simulink library "ADV_BF_MASTERbak"  (Simulink 8.6)
settings: Solver=VariableStepAuto  StartTime=0.0  StopTime=10.0  RelTol=1e-3
libraries: cdsEpicsOut x30, cdsFilt x17, cdsFiltCtrl x14, cdsTP x14, cdsEpicsIn x7, cdsMuxMatrix x3, VIS_LIB x2, cdsOsc x1, cdsEpicsBinIn x1, cdsFunctionCall x1, SIXOSEM_F_STAGE_MASTER x1
(part 1 of 3)
settings Model: Creator=controls  LastModifiedBy=controls

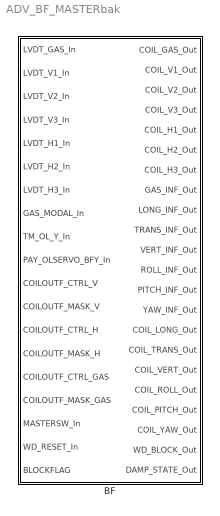
== system ADV_BF_MASTERbak ==
  BF : Subsystem

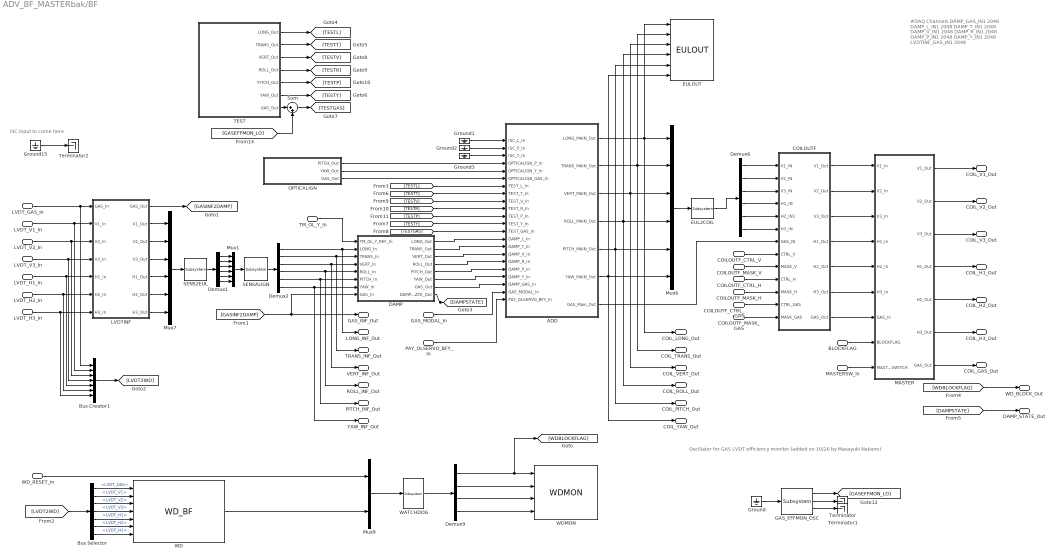
== system ADV_BF_MASTERbak/BF ==
  note: #DAQ Channels
      | DAMP_GAS_IN1 2048
      | DAMP_L_IN1 2048
      | DAMP_T_IN1 2048
      | DAMP_V_IN1 2048
      | DAMP_R_IN1 2048
      | DAMP_P_IN1 2048
      | DAMP_Y_IN1 2048
      | LVDTINF_GAS_IN1 2048
  note: ISC input to come here
  note: Oscillator for GAS LVDT efficiency monitor (added on 10/26 by Masayuki Nakano)
  LVDT_GAS_In : Inport
  LVDT_V1_In : Inport  Port=2
  LVDT_V2_In : Inport  Port=3
  LVDT_V3_In : Inport  Port=4
  LVDT_H1_In : Inport  Port=5
  LVDT_H2_In : Inport  Port=6
  LVDT_H3_In : Inport  Port=7
  GAS_MODAL_In : Inport  Port=8
  TM_OL_Y_In : Inport  Port=9
  PAY_OLSERVO_BFY_In : Inport  Port=10
  COILOUTF_CTRL_V : Inport  Port=11
  COILOUTF_MASK_V : Inport  Port=12
  COILOUTF_CTRL_H : Inport  Port=13
  COILOUTF_MASK_H : Inport  Port=14
  COILOUTF_CTRL_GAS : Inport  Port=15
  COILOUTF_MASK_GAS : Inport  Port=16
  MASTERSW_In : Inport  Port=17
  WD_RESET_In : Inport  Port=18
  BLOCKFLAG : Inport  Port=19
  ADD : Subsystem
  Bus Creator1 : BusCreator  Inputs='LVDT_GAS','LVDT_V1','LVDT_V2','LVDT_V3','LVDT_H1','LVDT_H2','LVDT_H3'
  Bus Selector : BusSelector  OutputSignals=LVDT_GAS,LVDT_V1,LVDT_V2,LVDT_V3,LVDT_H1,LVDT_H2,LVDT_H3
  COILOUTF : Subsystem
  DAMP : Subsystem
  Demux1 : Demux  Outputs=6
  Demux2 : Demux  Outputs=6
  Demux6 : Demux  Outputs=6
  Demux9 : Demux
  EUL2COIL : cdsMuxMatrix/Subsystem  Tag=cdsMuxMatrix  Description=|
      | ADL=SUS_INMATRIX.adl
      | SCRIPT=generate_KisselButton.py 4 5 #CHANNEL# > #TARGET_DIR#/#FULL_PART_NAME#_KB.adl
      settings: AttributesFormatString=%<Tag>
  EULOUT : VIS_LIB/EULOUT
  GAS_EFFMON_OSC : cdsOsc/Subsystem  Tag=cdsOsc  Description=Oscillator
      settings: AttributesFormatString=%<Tag>
  Ground{,1..3,15} (5 alike) : Ground
  LVDTINF : Subsystem
  MASTER : Subsystem
  Mux1 : Mux  Inputs=6
  Mux6 : Mux  Inputs=6
  Mux7 : Mux  Inputs=6
  Mux9 : Mux  Inputs=2
  OPTICALIGN : Subsystem
  SENS2EUL : cdsMuxMatrix/Subsystem  Tag=cdsMuxMatrix  Description=Any size matrix. Inputs and outputs must be connected using Mux and Demux parts.
      settings: AttributesFormatString=%<Tag>
  SENSALIGN : cdsMuxMatrix/Subsystem  Tag=cdsMuxMatrix  Description=Any size matrix. Inputs and outputs must be connected using Mux and Demux parts.
      settings: AttributesFormatString=%<Tag>
  Sum : Sum  Inputs=|++
  TEST : Subsystem
  Terminator : Terminator
  Terminator1 : Terminator
  Terminator2 : Terminator
  WATCHDOG : cdsFunctionCall/Subsystem  Tag=cdsFunctionCall  Description=inline OSEMWATCHDOG /opt/rtcds/userapps/release/vis/common/src/WATCHDOG.c
      settings: AttributesFormatString=%<Tag>\n%<Description>
  WD : VIS_LIB/WD_BF
  WDMON : SIXOSEM_F_STAGE_MASTER/SIXOSEM_F_STAGE_MASTER/WDMON
  COIL_GAS_Out : Outport
  COIL_V1_Out : Outport  Port=2
  COIL_V2_Out : Outport  Port=3
  COIL_V3_Out : Outport  Port=4
  COIL_H1_Out : Outport  Port=5
  COIL_H2_Out : Outport  Port=6
  COIL_H3_Out : Outport  Port=7
  GAS_INF_Out : Outport  Port=8
  LONG_INF_Out : Outport  Port=9
  TRANS_INF_Out : Outport  Port=10
  VERT_INF_Out : Outport  Port=11
  ROLL_INF_Out : Outport  Port=12
  PITCH_INF_Out : Outport  Port=13
  YAW_INF_Out : Outport  Port=14
  COIL_LONG_Out : Outport  Port=15
  COIL_TRANS_Out : Outport  Port=16
  COIL_VERT_Out : Outport  Port=17
  COIL_ROLL_Out : Outport  Port=18
  COIL_PITCH_Out : Outport  Port=19
  COIL_YAW_Out : Outport  Port=20
  WD_BLOCK_Out : Outport  Port=21
  DAMP_STATE_Out : Outport  Port=22
  wires:
  Ground15/1 -> Terminator2/1
  GAS_EFFMON_OSC/3 -> Terminator1/1
  GAS_EFFMON_OSC/2 -> Terminator/1
  Ground/1 -> GAS_EFFMON_OSC/1
  [GASEFFMON_LO] -> Sum/2
  Sum/1 -> [TESTGAS]
  TEST/7(GAS_Out) -> Sum/1
  GAS_EFFMON_OSC/1 -> [GASEFFMON_LO]
  COILOUTF_MASK_GAS/1 -> COILOUTF/13(MASK_GAS)
  COILOUTF_CTRL_GAS/1 -> COILOUTF/12(CTRL_GAS)
  COILOUTF_MASK_H/1 -> COILOUTF/11(MASK_H)
  COILOUTF_CTRL_H/1 -> COILOUTF/10(CTRL_H)
  LVDTINF/7(H3_Out) -> Mux7/6
  LVDTINF/6(H2_Out) -> Mux7/5
  LVDTINF/5(H1_Out) -> Mux7/4
  Bus Selector/7 -> WD/7  "<LVDT_H3>"
  Bus Selector/6 -> WD/6  "<LVDT_H2>"
  Bus Selector/5 -> WD/5  "<LVDT_H1>"
  Bus Selector/4 -> WD/4  "<LVDT_V3>"
  Bus Selector/3 -> WD/3  "<LVDT_V2>"
  Bus Selector/2 -> WD/2  "<LVDT_V1>"
  [DAMPSTATE] -> DAMP_STATE_Out/1
  [WDBLOCKFLAG] -> WD_BLOCK_Out/1
  MASTER/7(GAS_Out) -> COIL_GAS_Out/1
  MASTER/6(H3_Out) -> COIL_H3_Out/1
  MASTER/5(H2_Out) -> COIL_H2_Out/1
  MASTERSW_In/1 -> MASTER/9(MASTERSWITCH)
  BLOCKFLAG/1 -> MASTER/8(BLOCKFLAG)
  COILOUTF/4(H1_Out) -> MASTER/4(H1_In)
  COILOUTF/3(V3_Out) -> MASTER/3(V3_In)
  COILOUTF/2(V2_Out) -> MASTER/2(V2_In)
  COILOUTF/1(V1_Out) -> MASTER/1(V1_In)
  COILOUTF/7(GAS_Out) -> MASTER/7(GAS_In)
  COILOUTF/6(H3_Out) -> MASTER/6(H3_In)
  COILOUTF/5(H2_Out) -> MASTER/5(H2_In)
  Demux6/6 -> COILOUTF/6(H3_IN)
  Demux6/5 -> COILOUTF/5(H2_IN1)
  Demux6/4 -> COILOUTF/4(H1_IN)
  Demux6/3 -> COILOUTF/3(V3_IN)
  Demux6/2 -> COILOUTF/2(V2_IN)
  Demux6/1 -> COILOUTF/1(V1_IN)
  OPTICALIGN/3(GAS_Out) -> ADD/6(OPTICALIGN_GAS_In)
  OPTICALIGN/2(YAW_Out) -> ADD/5(OPTICALIGN_Y_In)
  OPTICALIGN/1(PITCH_Out) -> ADD/4(OPTICALIGN_P_In)
  ADD/1(LONG_MAIN_Out) -> EULOUT/1, COIL_LONG_Out/1, Mux6/1
  ADD/2(TRANS_MAIN_Out) -> EULOUT/2, COIL_TRANS_Out/1, Mux6/2
  ADD/3(VERT_MAIN_Out) -> EULOUT/3, COIL_VERT_Out/1, Mux6/3
  ADD/4(ROLL_MAIN_Out) -> EULOUT/4, COIL_ROLL_Out/1, Mux6/4
  ADD/5(PITCH_MAIN_Out) -> EULOUT/5, COIL_PITCH_Out/1, Mux6/5
  ADD/6(YAW_MAIN_Out) -> EULOUT/6, COIL_YAW_Out/1, Mux6/6
  ADD/7(GAS_Main_Out) -> COILOUTF/7(GAS_IN)
  DAMP/1(LONG_Out) -> ADD/14(DAMP_L_In)
  DAMP/2(TRANS_Out) -> ADD/15(DAMP_T_In)
  DAMP/3(VERT_Out) -> ADD/16(DAMP_V_In)
  DAMP/4(ROLL_Out) -> ADD/17(DAMP_R_In)
  DAMP/5(PITCH_Out) -> ADD/18(DAMP_P_In)
  DAMP/6(YAW_Out) -> ADD/19(DAMP_Y_In)
  DAMP/7(GAS_Out) -> ADD/20(DAMP_GAS_In)
  [TESTP] -> ADD/11(TEST_P_In)
  [TESTR] -> ADD/10(TEST_R_In)
  [TESTV] -> ADD/9(TEST_V_In)
  TEST/5(PITCH_Out) -> [TESTP]
  TEST/4(ROLL_Out) -> [TESTR]
  TEST/3(VERT_Out) -> [TESTV]
  DAMP/8(DAMP_STATE_Out) -> [DAMPSTATE]
  LVDTINF/4(V3_Out) -> Mux7/3
  LVDTINF/3(V2_Out) -> Mux7/2
  LVDTINF/2(V1_Out) -> Mux7/1
  SENSALIGN/1 -> Demux2/1
  Mux1/1 -> SENSALIGN/1
  Demux1/6 -> Mux1/6
  Demux1/5 -> Mux1/5
  Demux1/4 -> Mux1/4
  Demux1/3 -> Mux1/3
  Demux1/2 -> Mux1/2
  Demux1/1 -> Mux1/1
  SENS2EUL/1 -> Demux1/1
  Demux2/1 -> LONG_INF_Out/1, DAMP/2(LONG_In)
  Bus Selector/1 -> WD/1  "<LVDT_GAS>"
  MASTER/4(H1_Out) -> COIL_H1_Out/1
  [TESTGAS] -> ADD/13(TEST_GAS_In)
  [TESTY] -> ADD/12(TEST_Y_In)
  [TESTT] -> ADD/8(TEST_T_In)
  [TESTL] -> ADD/7(TEST_L_In)
  TEST/6(YAW_Out) -> [TESTY]
  TEST/2(TRANS_Out) -> [TESTT]
  TEST/1(LONG_Out) -> [TESTL]
  LVDTINF/1(GAS_Out) -> [GASINF2DAMP]
  LVDT_GAS_In/1 -> LVDTINF/1(GAS_In), Bus Creator1/1
  COILOUTF_MASK_V/1 -> COILOUTF/9(MASK_V)
  COILOUTF_CTRL_V/1 -> COILOUTF/8(CTRL_V)
  Bus Creator1/1 -> [LVDT2WD]
  LVDT_H3_In/1 -> Bus Creator1/7, LVDTINF/7(H3_In)
  LVDT_H2_In/1 -> Bus Creator1/6, LVDTINF/6(H2_In)
  LVDT_H1_In/1 -> Bus Creator1/5, LVDTINF/5(H1_In)
  LVDT_V3_In/1 -> LVDTINF/4(V3_In), Bus Creator1/4
  LVDT_V2_In/1 -> LVDTINF/3(V2_In), Bus Creator1/3
  LVDT_V1_In/1 -> LVDTINF/2(V1_In), Bus Creator1/2
  WATCHDOG/1 -> Demux9/1
  Mux9/1 -> WATCHDOG/1
  Demux9/4 -> WDMON/4
  Demux9/3 -> WDMON/3
  Demux9/2 -> WDMON/2
  Demux9/1 -> WDMON/1, [WDBLOCKFLAG]
  [LVDT2WD] -> Bus Selector/1
  WD/1 -> Mux9/2
  WD_RESET_In/1 -> Mux9/1
  MASTER/3(V3_Out) -> COIL_V3_Out/1
  MASTER/2(V2_Out) -> COIL_V2_Out/1
  MASTER/1(V1_Out) -> COIL_V1_Out/1
  EUL2COIL/1 -> Demux6/1
  Mux6/1 -> EUL2COIL/1
  Mux7/1 -> SENS2EUL/1
  GAS_MODAL_In/1 -> ADD/21(GAS_MODAL_In)
  TM_OL_Y_In/1 -> DAMP/1(TM_OL_Y_REF_In)
  Ground1/1 -> ADD/1(ISC_L_In)
  Ground2/1 -> ADD/2(ISC_P_In)
  Ground3/1 -> ADD/3(ISC_Y_In)
  PAY_OLSERVO_BFY_In/1 -> ADD/22(PAY_OLSERVO_BFY_In)
  Demux2/6 -> YAW_INF_Out/1, DAMP/7(YAW_In)
  Demux2/4 -> ROLL_INF_Out/1, DAMP/5(ROLL_In)
  Demux2/2 -> TRANS_INF_Out/1, DAMP/3(TRANS_In)
  Demux2/5 -> PITCH_INF_Out/1, DAMP/6(PITCH_In)
  Demux2/3 -> VERT_INF_Out/1, DAMP/4(VERT_In)
  [GASINF2DAMP] -> GAS_INF_Out/1, DAMP/8(GAS_In)

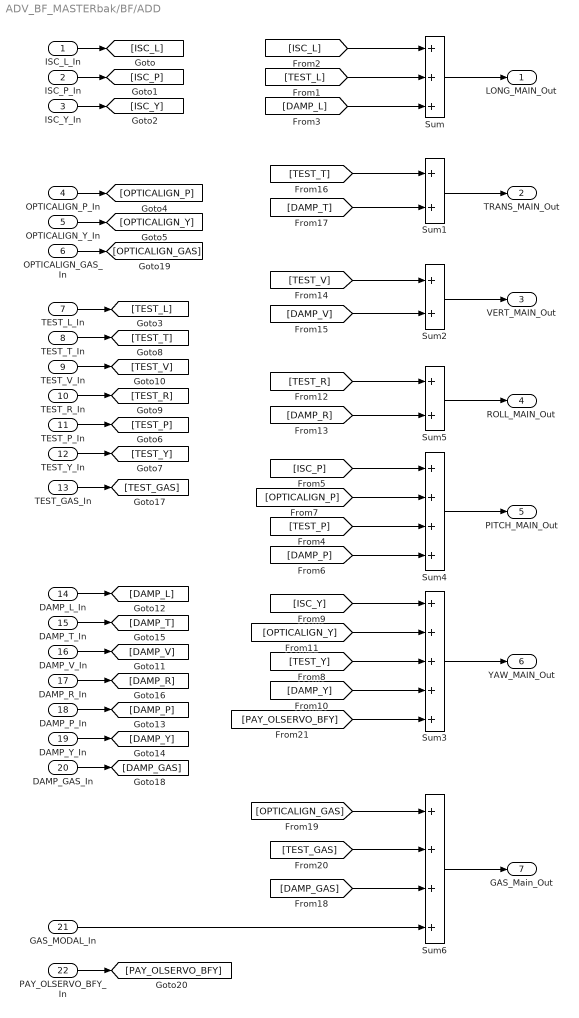
== system ADV_BF_MASTERbak/BF/ADD ==
  ISC_L_In : Inport
  ISC_P_In : Inport  Port=2
  ISC_Y_In : Inport  Port=3
  OPTICALIGN_P_In : Inport  Port=4
  OPTICALIGN_Y_In : Inport  Port=5
  OPTICALIGN_GAS_In : Inport  Port=6
  TEST_L_In : Inport  Port=7
  TEST_T_In : Inport  Port=8
  TEST_V_In : Inport  Port=9
  TEST_R_In : Inport  Port=10
  TEST_P_In : Inport  Port=11
  TEST_Y_In : Inport  Port=12
  TEST_GAS_In : Inport  Port=13
  DAMP_L_In : Inport  Port=14
  DAMP_T_In : Inport  Port=15
  DAMP_V_In : Inport  Port=16
  DAMP_R_In : Inport  Port=17
  DAMP_P_In : Inport  Port=18
  DAMP_Y_In : Inport  Port=19
  DAMP_GAS_In : Inport  Port=20
  GAS_MODAL_In : Inport  Port=21
  PAY_OLSERVO_BFY_In : Inport  Port=22
  Sum : Sum  Inputs=+++
  Sum1 : Sum
  Sum2 : Sum
  Sum3 : Sum  Inputs=+++++
  Sum4 : Sum  Inputs=++++
  Sum5 : Sum
  Sum6 : Sum  Inputs=++++
  LONG_MAIN_Out : Outport
  TRANS_MAIN_Out : Outport  Port=2
  VERT_MAIN_Out : Outport  Port=3
  ROLL_MAIN_Out : Outport  Port=4
  PITCH_MAIN_Out : Outport  Port=5
  YAW_MAIN_Out : Outport  Port=6
  GAS_Main_Out : Outport  Port=7
  wires:
  [DAMP_GAS] -> Sum6/3
  [TEST_GAS] -> Sum6/2
  [OPTICALIGN_GAS] -> Sum6/1
  DAMP_GAS_In/1 -> [DAMP_GAS]
  DAMP_Y_In/1 -> [DAMP_Y]
  DAMP_P_In/1 -> [DAMP_P]
  DAMP_R_In/1 -> [DAMP_R]
  DAMP_V_In/1 -> [DAMP_V]
  DAMP_T_In/1 -> [DAMP_T]
  DAMP_L_In/1 -> [DAMP_L]
  TEST_GAS_In/1 -> [TEST_GAS]
  TEST_Y_In/1 -> [TEST_Y]
  TEST_P_In/1 -> [TEST_P]
  TEST_R_In/1 -> [TEST_R]
  TEST_V_In/1 -> [TEST_V]
  TEST_T_In/1 -> [TEST_T]
  TEST_L_In/1 -> [TEST_L]
  OPTICALIGN_GAS_In/1 -> [OPTICALIGN_GAS]
  Sum6/1 -> GAS_Main_Out/1
  Sum4/1 -> PITCH_MAIN_Out/1
  Sum3/1 -> YAW_MAIN_Out/1
  Sum/1 -> LONG_MAIN_Out/1
  [ISC_L] -> Sum/1
  [TEST_L] -> Sum/2
  [DAMP_L] -> Sum/3
  Sum5/1 -> ROLL_MAIN_Out/1
  Sum2/1 -> VERT_MAIN_Out/1
  Sum1/1 -> TRANS_MAIN_Out/1
  OPTICALIGN_P_In/1 -> [OPTICALIGN_P]
  OPTICALIGN_Y_In/1 -> [OPTICALIGN_Y]
  ISC_L_In/1 -> [ISC_L]
  ISC_P_In/1 -> [ISC_P]
  ISC_Y_In/1 -> [ISC_Y]
  [ISC_P] -> Sum4/1
  [OPTICALIGN_P] -> Sum4/2
  [TEST_P] -> Sum4/3
  [DAMP_P] -> Sum4/4
  [ISC_Y] -> Sum3/1
  [OPTICALIGN_Y] -> Sum3/2
  [TEST_Y] -> Sum3/3
  [DAMP_Y] -> Sum3/4
  [TEST_R] -> Sum5/1
  [DAMP_R] -> Sum5/2
  [TEST_T] -> Sum1/1
  [DAMP_T] -> Sum1/2
  [TEST_V] -> Sum2/1
  [DAMP_V] -> Sum2/2
  GAS_MODAL_In/1 -> Sum6/4
  PAY_OLSERVO_BFY_In/1 -> [PAY_OLSERVO_BFY]
  [PAY_OLSERVO_BFY] -> Sum3/5

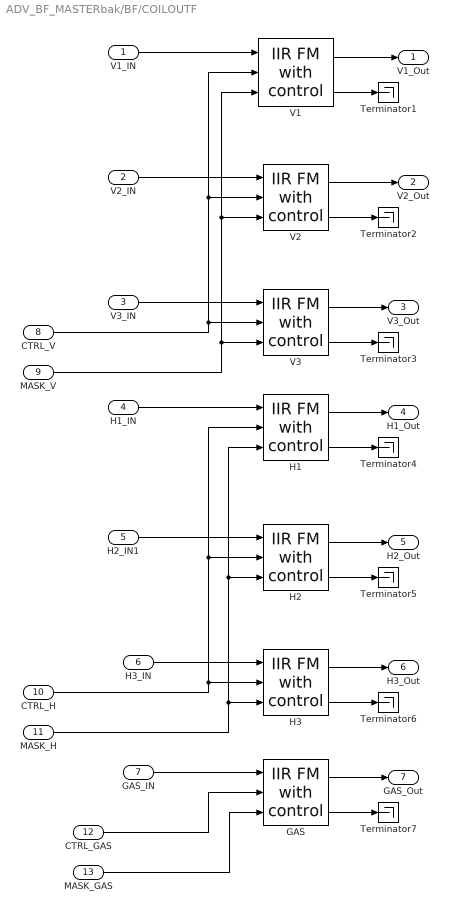
== system ADV_BF_MASTERbak/BF/COILOUTF ==
  V1_IN : Inport
  V2_IN : Inport  Port=2
  V3_IN : Inport  Port=3
  H1_IN : Inport  Port=4
  H2_IN1 : Inport  Port=5
  H3_IN : Inport  Port=6
  GAS_IN : Inport  Port=7
  CTRL_V : Inport  Port=8
  MASK_V : Inport  Port=9
  CTRL_H : Inport  Port=10
  MASK_H : Inport  Port=11
  CTRL_GAS : Inport  Port=12
  MASK_GAS : Inport  Port=13
  GAS : cdsFiltCtrl/IIR FM with control  Tag=cdsFiltCtrl  Description=|
      | cdsFiltCntrl is the standard IIR filter module (exactly the same as cdsFilt) but with added control data output 'Ctrl'. Filter module digital signal output appears on the first output, which is called 'Val'. 'Ctrl' output has a bit pattern encoding the state of filter's on/off switches (FM1 through FM10). The bit values are:
      |                                                                                                                                                                                                                                                                                                                                       
      | module 	hex	dec                                                                                                                                                                                                                                                                                                                       
      | -----------------------                                                                                                                                                                                                                                                                                                               
      | FM1	0x20                    32                                                                                                                                                                                                                                                                                                        
      | FM2	0x80                     128                                                                                                                                                                                                                                                                                                      
      | FM3	0x200                   512                                                                                                                                                                                                                                                                                                       
      | FM4	0x800                   2048                                                                                                                                                                                                                                                                                                      
      | FM5	0x2000                 8192                                                                                                                                                                                                                                                                                                       
      | FM6	0x8000                 32768                                                                                                                                                                                                                                                                                                      
      | FM7	0x20000                131072                                                                                                                                                                                                                                                                                                     
      | FM8	0x80000                 524288                                                                                                                                                                                                                                                                                                    
      | FM9	0x200000               2097152                                                                                                                                                                                                                                                                                                    
      | FM10	0x800000               8388608                                                                                                                                                                                                                                                                                                   
      |                                                                                                                                                                                                                                                                                                                                       
      | This bit data can be used to drive some other switches or it can be output using a binary I/O module.
      settings: AttributesFormatString=%<Tag>
  H1 : cdsFiltCtrl/IIR FM with control  Tag=cdsFiltCtrl  Description=|
      | cdsFiltCntrl is the standard IIR filter module (exactly the same as cdsFilt) but with added control data output 'Ctrl'. Filter module digital signal output appears on the first output, which is called 'Val'. 'Ctrl' output has a bit pattern encoding the state of filter's on/off switches (FM1 through FM10). The bit values are:
      |                                                                                                                                                                                                                                                                                                                                       
      | module 	hex	dec                                                                                                                                                                                                                                                                                                                       
      | -----------------------                                                                                                                                                                                                                                                                                                               
      | FM1	0x20                    32                                                                                                                                                                                                                                                                                                        
      | FM2	0x80                     128                                                                                                                                                                                                                                                                                                      
      | FM3	0x200                   512                                                                                                                                                                                                                                                                                                       
      | FM4	0x800                   2048                                                                                                                                                                                                                                                                                                      
      | FM5	0x2000                 8192                                                                                                                                                                                                                                                                                                       
      | FM6	0x8000                 32768                                                                                                                                                                                                                                                                                                      
      | FM7	0x20000                131072                                                                                                                                                                                                                                                                                                     
      | FM8	0x80000                 524288                                                                                                                                                                                                                                                                                                    
      | FM9	0x200000               2097152                                                                                                                                                                                                                                                                                                    
      | FM10	0x800000               8388608                                                                                                                                                                                                                                                                                                   
      |                                                                                                                                                                                                                                                                                                                                       
      | This bit data can be used to drive some other switches or it can be output using a binary I/O module.
      settings: AttributesFormatString=%<Tag>
  H2 : cdsFiltCtrl/IIR FM with control  Tag=cdsFiltCtrl  Description=|
      | cdsFiltCntrl is the standard IIR filter module (exactly the same as cdsFilt) but with added control data output 'Ctrl'. Filter module digital signal output appears on the first output, which is called 'Val'. 'Ctrl' output has a bit pattern encoding the state of filter's on/off switches (FM1 through FM10). The bit values are:
      |                                                                                                                                                                                                                                                                                                                                       
      | module 	hex	dec                                                                                                                                                                                                                                                                                                                       
      | -----------------------                                                                                                                                                                                                                                                                                                               
      | FM1	0x20                    32                                                                                                                                                                                                                                                                                                        
      | FM2	0x80                     128                                                                                                                                                                                                                                                                                                      
      | FM3	0x200                   512                                                                                                                                                                                                                                                                                                       
      | FM4	0x800                   2048                                                                                                                                                                                                                                                                                                      
      | FM5	0x2000                 8192                                                                                                                                                                                                                                                                                                       
      | FM6	0x8000                 32768                                                                                                                                                                                                                                                                                                      
      | FM7	0x20000                131072                                                                                                                                                                                                                                                                                                     
      | FM8	0x80000                 524288                                                                                                                                                                                                                                                                                                    
      | FM9	0x200000               2097152                                                                                                                                                                                                                                                                                                    
      | FM10	0x800000               8388608                                                                                                                                                                                                                                                                                                   
      |                                                                                                                                                                                                                                                                                                                                       
      | This bit data can be used to drive some other switches or it can be output using a binary I/O module.
      settings: AttributesFormatString=%<Tag>
  H3 : cdsFiltCtrl/IIR FM with control  Tag=cdsFiltCtrl  Description=|
      | cdsFiltCntrl is the standard IIR filter module (exactly the same as cdsFilt) but with added control data output 'Ctrl'. Filter module digital signal output appears on the first output, which is called 'Val'. 'Ctrl' output has a bit pattern encoding the state of filter's on/off switches (FM1 through FM10). The bit values are:
      |                                                                                                                                                                                                                                                                                                                                       
      | module 	hex	dec                                                                                                                                                                                                                                                                                                                       
      | -----------------------                                                                                                                                                                                                                                                                                                               
      | FM1	0x20                    32                                                                                                                                                                                                                                                                                                        
      | FM2	0x80                     128                                                                                                                                                                                                                                                                                                      
      | FM3	0x200                   512                                                                                                                                                                                                                                                                                                       
      | FM4	0x800                   2048                                                                                                                                                                                                                                                                                                      
      | FM5	0x2000                 8192                                                                                                                                                                                                                                                                                                       
      | FM6	0x8000                 32768                                                                                                                                                                                                                                                                                                      
      | FM7	0x20000                131072                                                                                                                                                                                                                                                                                                     
      | FM8	0x80000                 524288                                                                                                                                                                                                                                                                                                    
      | FM9	0x200000               2097152                                                                                                                                                                                                                                                                                                    
      | FM10	0x800000               8388608                                                                                                                                                                                                                                                                                                   
      |                                                                                                                                                                                                                                                                                                                                       
      | This bit data can be used to drive some other switches or it can be output using a binary I/O module.
      settings: AttributesFormatString=%<Tag>
  Terminator{1..7} (7 alike) : Terminator
  V1 : cdsFiltCtrl/IIR FM with control  Tag=cdsFiltCtrl  Description=|
      | cdsFiltCntrl is the standard IIR filter module (exactly the same as cdsFilt) but with added control data output 'Ctrl'. Filter module digital signal output appears on the first output, which is called 'Val'. 'Ctrl' output has a bit pattern encoding the state of filter's on/off switches (FM1 through FM10). The bit values are:
      |                                                                                                                                                                                                                                                                                                                                       
      | module 	hex	dec                                                                                                                                                                                                                                                                                                                       
      | -----------------------                                                                                                                                                                                                                                                                                                               
      | FM1	0x20                    32                                                                                                                                                                                                                                                                                                        
      | FM2	0x80                     128                                                                                                                                                                                                                                                                                                      
      | FM3	0x200                   512                                                                                                                                                                                                                                                                                                       
      | FM4	0x800                   2048                                                                                                                                                                                                                                                                                                      
      | FM5	0x2000                 8192                                                                                                                                                                                                                                                                                                       
      | FM6	0x8000                 32768                                                                                                                                                                                                                                                                                                      
      | FM7	0x20000                131072                                                                                                                                                                                                                                                                                                     
      | FM8	0x80000                 524288                                                                                                                                                                                                                                                                                                    
      | FM9	0x200000               2097152                                                                                                                                                                                                                                                                                                    
      | FM10	0x800000               8388608                                                                                                                                                                                                                                                                                                   
      |                                                                                                                                                                                                                                                                                                                                       
      | This bit data can be used to drive some other switches or it can be output using a binary I/O module.
      settings: AttributesFormatString=%<Tag>
  V2 : cdsFiltCtrl/IIR FM with control  Tag=cdsFiltCtrl  Description=|
      | cdsFiltCntrl is the standard IIR filter module (exactly the same as cdsFilt) but with added control data output 'Ctrl'. Filter module digital signal output appears on the first output, which is called 'Val'. 'Ctrl' output has a bit pattern encoding the state of filter's on/off switches (FM1 through FM10). The bit values are:
      |                                                                                                                                                                                                                                                                                                                                       
      | module 	hex	dec                                                                                                                                                                                                                                                                                                                       
      | -----------------------                                                                                                                                                                                                                                                                                                               
      | FM1	0x20                    32                                                                                                                                                                                                                                                                                                        
      | FM2	0x80                     128                                                                                                                                                                                                                                                                                                      
      | FM3	0x200                   512                                                                                                                                                                                                                                                                                                       
      | FM4	0x800                   2048                                                                                                                                                                                                                                                                                                      
      | FM5	0x2000                 8192                                                                                                                                                                                                                                                                                                       
      | FM6	0x8000                 32768                                                                                                                                                                                                                                                                                                      
      | FM7	0x20000                131072                                                                                                                                                                                                                                                                                                     
      | FM8	0x80000                 524288                                                                                                                                                                                                                                                                                                    
      | FM9	0x200000               2097152                                                                                                                                                                                                                                                                                                    
      | FM10	0x800000               8388608                                                                                                                                                                                                                                                                                                   
      |                                                                                                                                                                                                                                                                                                                                       
      | This bit data can be used to drive some other switches or it can be output using a binary I/O module.
      settings: AttributesFormatString=%<Tag>
  V3 : cdsFiltCtrl/IIR FM with control  Tag=cdsFiltCtrl  Description=|
      | cdsFiltCntrl is the standard IIR filter module (exactly the same as cdsFilt) but with added control data output 'Ctrl'. Filter module digital signal output appears on the first output, which is called 'Val'. 'Ctrl' output has a bit pattern encoding the state of filter's on/off switches (FM1 through FM10). The bit values are:
      |                                                                                                                                                                                                                                                                                                                                       
      | module 	hex	dec                                                                                                                                                                                                                                                                                                                       
      | -----------------------                                                                                                                                                                                                                                                                                                               
      | FM1	0x20                    32                                                                                                                                                                                                                                                                                                        
      | FM2	0x80                     128                                                                                                                                                                                                                                                                                                      
      | FM3	0x200                   512                                                                                                                                                                                                                                                                                                       
      | FM4	0x800                   2048                                                                                                                                                                                                                                                                                                      
      | FM5	0x2000                 8192                                                                                                                                                                                                                                                                                                       
      | FM6	0x8000                 32768                                                                                                                                                                                                                                                                                                      
      | FM7	0x20000                131072                                                                                                                                                                                                                                                                                                     
      | FM8	0x80000                 524288                                                                                                                                                                                                                                                                                                    
      | FM9	0x200000               2097152                                                                                                                                                                                                                                                                                                    
      | FM10	0x800000               8388608                                                                                                                                                                                                                                                                                                   
      |                                                                                                                                                                                                                                                                                                                                       
      | This bit data can be used to drive some other switches or it can be output using a binary I/O module.
      settings: AttributesFormatString=%<Tag>
  V1_Out : Outport
  V2_Out : Outport  Port=2
  V3_Out : Outport  Port=3
  H1_Out : Outport  Port=4
  H2_Out : Outport  Port=5
  H3_Out : Outport  Port=6
  GAS_Out : Outport  Port=7
  wires:
  MASK_GAS/1 -> GAS/3
  CTRL_GAS/1 -> GAS/2
  MASK_H/1 -> H2/3, H1/3, H3/3
  CTRL_H/1 -> H2/2, H1/2, H3/2
  MASK_V/1 -> V3/3, V2/3, V1/3
  CTRL_V/1 -> V3/2, V2/2, V1/2
  H3_IN/1 -> H3/1
  H2_IN1/1 -> H2/1
  H1_IN/1 -> H1/1
  V3_IN/1 -> V3/1
  V2_IN/1 -> V2/1
  V1_IN/1 -> V1/1
  GAS/2 -> Terminator7/1
  GAS_IN/1 -> GAS/1
  GAS/1 -> GAS_Out/1
  H3/2 -> Terminator6/1
  H3/1 -> H3_Out/1
  H2/2 -> Terminator5/1
  H2/1 -> H2_Out/1
  H1/2 -> Terminator4/1
  H1/1 -> H1_Out/1
  V1/2 -> Terminator1/1
  V2/2 -> Terminator2/1
  V3/2 -> Terminator3/1
  V1/1 -> V1_Out/1
  V2/1 -> V2_Out/1
  V3/1 -> V3_Out/1
